simulink model "Driver3"  (R2023b)
settings: Solver=VariableStepAuto  StartTime=0.0  StopTime=10.0  RelTol=1e-3
settings Model: Creator=user  LastModifiedBy=user

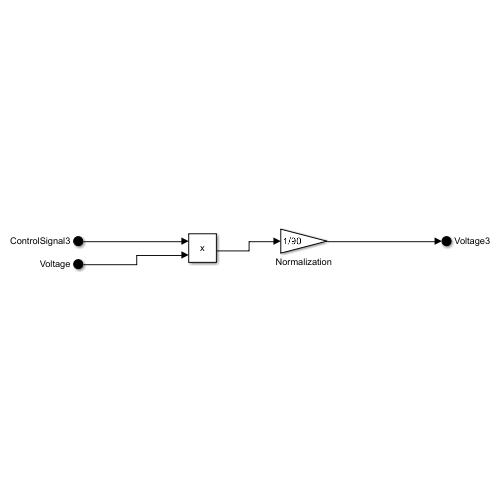
[thumbnail: Simulink's stored preview of the top-level diagram]
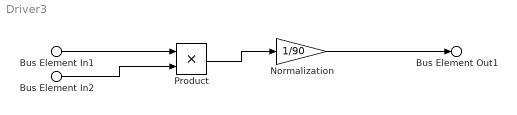
== system Driver3 ==
  Bus Element In1 : Inport  PortName=ControlSignal3
  Bus Element In2 : Inport  Port=2  PortName=Voltage
  Normalization : Gain  Gain=1/90
  Product : Product
  Bus Element Out1 : Outport  PortName=Voltage3
  wires:
  Normalization/1 -> Bus Element Out1/1
  Bus Element In2/1 -> Product/2
  Product/1 -> Normalization/1
  Bus Element In1/1 -> Product/1
